simulink model "platoon"  (R2024b)
settings: Solver=FixedStepAuto  StartTime=0.0  StopTime=20  RelTol=1e-3
libraries: slpidlib x2
settings Model: Creator=Corné  LastModifiedBy=Corné

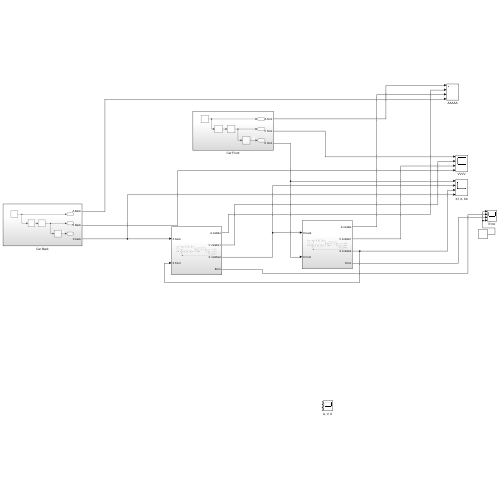
[thumbnail: Simulink's stored preview of the top-level diagram]
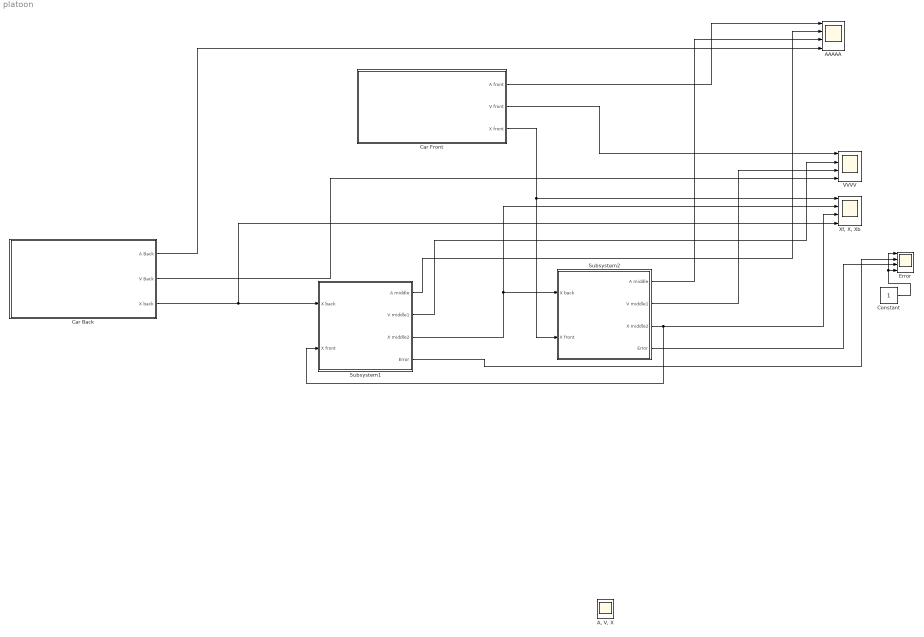
== system platoon ==
  "A, V, X " : Scope  NumInputPorts=3
  AAAAA : Scope  NumInputPorts=4
  Car Back : Subsystem
  Car Front : Subsystem
  Constant : Constant
  Error : Scope  NumInputPorts=4
  Subsystem1 : Subsystem
  Subsystem2 : Subsystem
  VVVV : Scope  NumInputPorts=4
  "Xf, X, Xb" : Scope  NumInputPorts=4
  wires:
  Car Back/3(X back) -> "Xf, X, Xb"/4, Subsystem1/1("X back ")
  Car Front/3(X front) -> Subsystem2/2(X front), "Xf, X, Xb"/1
  Subsystem1/4(Error) -> Error/2
  Subsystem1/3(X middle2) -> "Xf, X, Xb"/2, Subsystem2/1("X back ")
  Subsystem2/3(X middle2) -> "Xf, X, Xb"/3, Subsystem1/2(X front)
  Subsystem2/4(Error) -> Error/3
  Car Front/1(A front) -> AAAAA/1
  Car Back/1(A Back) -> AAAAA/4
  Subsystem1/1(A middle) -> AAAAA/2
  Subsystem2/1(A middle) -> AAAAA/3
  Car Front/2(V front) -> VVVV/1
  Car Back/2(V Back) -> VVVV/4
  Subsystem1/2(V middle1) -> VVVV/2
  Subsystem2/2(V middle1) -> VVVV/3
  Constant/1 -> Error/4, Error/1

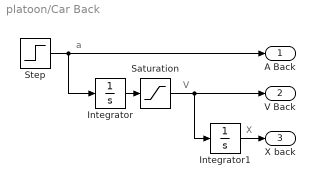
== system platoon/Car Back ==
  note: X
  note: V
  note: a
  Integrator : Integrator  InitialCondition=30
  Integrator1 : Integrator
  Saturation : Saturate  UpperLimit=30  LowerLimit=-50
  Step : Step  Time=0  After=0  SampleTime=0
  A Back : Outport
  V Back : Outport  Port=2
  X back : Outport  Port=3
  wires:
  Integrator/1 -> Saturation/1
  Step/1 -> Integrator/1, A Back/1
  Integrator1/1 -> X back/1
  Saturation/1 -> Integrator1/1, V Back/1

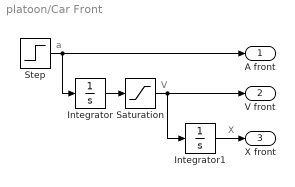
== system platoon/Car Front ==
  note: X
  note: V
  note: a
  Integrator : Integrator  InitialCondition=30
  Integrator1 : Integrator  InitialCondition=12*3
  Saturation : Saturate  UpperLimit=30  LowerLimit=-50
  Step : Step  Time=0  After=0  SampleTime=0
  A front : Outport
  V front : Outport  Port=2
  X front : Outport  Port=3
  wires:
  Integrator/1 -> Saturation/1
  Step/1 -> A front/1, Integrator/1
  Integrator1/1 -> X front/1
  Saturation/1 -> V front/1, Integrator1/1

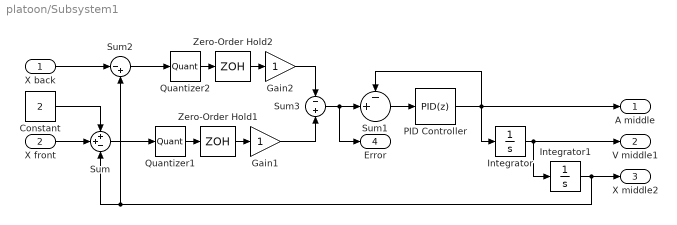
== system platoon/Subsystem1 ==
  "X back " : Inport
  X front : Inport  Port=2
  Constant : Constant  Value=2
  Gain1 : Gain
  Gain2 : Gain
  Integrator : Integrator  InitialCondition=22
  Integrator1 : Integrator  InitialCondition=10
  PID Controller : slpidlib/PID Controller  Controller=PID  Form=Parallel  TimeDomain=Discrete-time  UseExternalTs=off  SampleTime=-1  IntegratorMethod=Forward Euler  FilterMethod=Forward Euler  ControllerParametersSource=internal  P=0.2  I=0  UseKiTs=off  D=0.6  UseExternalDerivativeSource=off  N=100  UseFilter=on  TunerSelectOption=Transfer Function Based (PID Tuner App)  InitialConditionSource=internal  InitialConditionForIntegrator=0  InitialConditionForFilter=0  DifferentiatorICPrevScaledInput=0  ExternalReset=none  TrackingMode=off  Kt=1  LimitOutput=off  SatLimitsSource=internal  UpperSaturationLimit=inf  LowerSaturationLimit=-inf  LinearizeAsGain=on  AntiWindupMode=none  Kb=1  LimitIntegrator=off  UpperIntegratorSaturationLimit=inf  LowerIntegratorSaturationLimit=-inf  POutMin=[]  POutMax=[]  IOutMin=[]  IOutMax=[]  DOutMin=[]  DOutMax=[]  NOutMin=[]  NOutMax=[]  SumOutMin=[]  SumOutMax=[]  SaturationOutMin=[]  SaturationOutMax=[]  PParamMin=[]  PParamMax=[]  IParamMin=[]  IParamMax=[]  DParamMin=[]  DParamMax=[]  NParamMin=[]  NParamMax=[]  KbParamMin=[]  KbParamMax=[]  KtParamMin=[]  KtParamMax=[]  KbOutMin=[]  KbOutMax=[]  KtOutMin=[]  KtOutMax=[]  IntegratorOutMin=[]  IntegratorOutMax=[]  FilterOutMin=[]  FilterOutMax=[]  SumI1OutMin=[]  SumI1OutMax=[]  SumI2OutMin=[]  SumI2OutMax=[]  SumI3OutMin=[]  SumI3OutMax=[]  SumI4OutMin=[]  SumI4OutMax=[]  SumDOutMin=[]  SumDOutMax=[]  DifferentiatorOutMin=[]  DifferentiatorOutMax=[]  FilterDiffOutCoefMin=[]  FilterDiffOutCoefMax=[]  ReciprocalOutMin=[]  ReciprocalOutMax=[]  SumDenOutMin=[]  SumDenOutMax=[]  SumNumOutMin=[]  SumNumOutMax=[]  DivideOutMin=[]  DivideOutMax=[]  UdiffTsProdOutMin=[]  UdiffTsProdOutMax=[]  NTsProdOutMin=[]  NTsProdOutMax=[]  UintegralTsProdOutMin=[]  UintegralTsProdOutMax=[]  UngainTsProdOutMin=[]  UngainTsProdOutMax=[]  ClampingZeroOutDataTypeStr=Inherit: Inherit via back propagation  ClampingZeroOutMin=[]  ClampingZeroOutMax=[]  FilterDenConstantOutDataTypeStr=Inherit: Inherit via back propagation  FilterDenConstantOutMin=[]  FilterDenConstantOutMax=[]  PCopyOutDataTypeStr=Inherit: Inherit via back propagation  PCopyOutMin=[]  PCopyOutMax=[]  NCopyOutDataTypeStr=Inherit: Inherit via back propagation  NCopyOutMin=[]  NCopyOutMax=[]  IntegratorContinuousStateAttributes=''  IntegratorStateMustResolveToSignalObject=off  IntegratorRTWStateStorageClass=Auto  FilterContinuousStateAttributes=''  FilterStateMustResolveToSignalObject=off  FilterRTWStateStorageClass=Auto  ParallelPVariant=InternalParameters  IdealPVariant=Disabled  IVariant=InternalParameters  DVariant=InternalParameters  IntegratorVariant=Discrete  SatVariant=Disabled  AWVariant=Passthrough  PCopyVariant=Disabled  TRVariant=Disabled  FdbkBlocksVariant=Forward  IdealPFdbkVariant=Disabled  SatFdbkVariant=Disabled  DerivativeFilterVariant=ForwardEulerFilter  NVariant=InternalParameters  NCopyVariant=Disabled  FilterICVariant=InternalICsFilter  IntegratorICVariant=InternalICs  ExternalResetVariant=Disabled  TRSumVariant=Passthrough  SumFdbkVariant=Disabled  SumVariant=Sum_PID  TsampFilterVariant=InternalTs  TsampNgainVariant=Passthrough  TsampIntegralVariant=Disabled_SignalSpec  ExternalSaturationOutDataTypeStr=Inherit: Same as second input  DerivativeSourceVariant=ErrorSignal  PreIntVariant=InternalPreInt
  Quantizer1 : Quantizer  QuantizationInterval=0.1
  Quantizer2 : Quantizer  QuantizationInterval=0.1
  Sum : Sum  Inputs=++-
  Sum1 : Sum  Inputs=-+|
  Sum2 : Sum  Inputs=|-+
  Sum3 : Sum  Inputs=-|+
  Zero-Order Hold1 : ZeroOrderHold  SampleTime=0.1
  Zero-Order Hold2 : ZeroOrderHold  SampleTime=0.1
  A middle : Outport
  V middle1 : Outport  Port=2
  X middle2 : Outport  Port=3
  Error : Outport  Port=4
  wires:
  Integrator/1 -> Integrator1/1, V middle1/1
  Integrator1/1 -> Sum2/2, Sum/3, X middle2/1
  Sum1/1 -> PID Controller/1
  PID Controller/1 -> Sum1/1, Integrator/1, A middle/1
  X front/1 -> Sum/2
  Sum3/1 -> Error/1, Sum1/2
  Quantizer1/1 -> Zero-Order Hold1/1
  Zero-Order Hold1/1 -> Gain1/1
  Sum/1 -> Quantizer1/1
  Gain1/1 -> Sum3/2
  Quantizer2/1 -> Zero-Order Hold2/1
  Zero-Order Hold2/1 -> Gain2/1
  Sum2/1 -> Quantizer2/1
  Gain2/1 -> Sum3/1
  Constant/1 -> Sum/1
  "X back "/1 -> Sum2/1

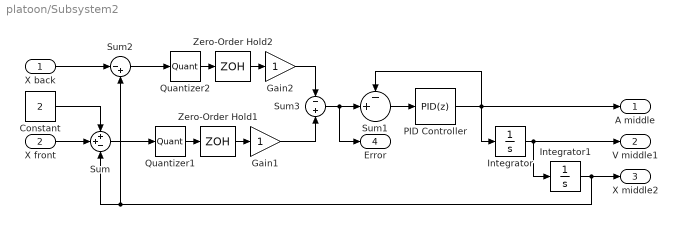
== system platoon/Subsystem2 ==
  "X back " : Inport
  X front : Inport  Port=2
  Constant : Constant  Value=2
  Gain1 : Gain
  Gain2 : Gain
  Integrator : Integrator  InitialCondition=22
  Integrator1 : Integrator  InitialCondition=20
  PID Controller : slpidlib/PID Controller  Controller=PID  Form=Parallel  TimeDomain=Discrete-time  UseExternalTs=off  SampleTime=-1  IntegratorMethod=Forward Euler  FilterMethod=Forward Euler  ControllerParametersSource=internal  P=0.2  I=0  UseKiTs=off  D=0.6  UseExternalDerivativeSource=off  N=100  UseFilter=on  TunerSelectOption=Transfer Function Based (PID Tuner App)  InitialConditionSource=internal  InitialConditionForIntegrator=0  InitialConditionForFilter=0  DifferentiatorICPrevScaledInput=0  ExternalReset=none  TrackingMode=off  Kt=1  LimitOutput=off  SatLimitsSource=internal  UpperSaturationLimit=inf  LowerSaturationLimit=-inf  LinearizeAsGain=on  AntiWindupMode=none  Kb=1  LimitIntegrator=off  UpperIntegratorSaturationLimit=inf  LowerIntegratorSaturationLimit=-inf  POutMin=[]  POutMax=[]  IOutMin=[]  IOutMax=[]  DOutMin=[]  DOutMax=[]  NOutMin=[]  NOutMax=[]  SumOutMin=[]  SumOutMax=[]  SaturationOutMin=[]  SaturationOutMax=[]  PParamMin=[]  PParamMax=[]  IParamMin=[]  IParamMax=[]  DParamMin=[]  DParamMax=[]  NParamMin=[]  NParamMax=[]  KbParamMin=[]  KbParamMax=[]  KtParamMin=[]  KtParamMax=[]  KbOutMin=[]  KbOutMax=[]  KtOutMin=[]  KtOutMax=[]  IntegratorOutMin=[]  IntegratorOutMax=[]  FilterOutMin=[]  FilterOutMax=[]  SumI1OutMin=[]  SumI1OutMax=[]  SumI2OutMin=[]  SumI2OutMax=[]  SumI3OutMin=[]  SumI3OutMax=[]  SumI4OutMin=[]  SumI4OutMax=[]  SumDOutMin=[]  SumDOutMax=[]  DifferentiatorOutMin=[]  DifferentiatorOutMax=[]  FilterDiffOutCoefMin=[]  FilterDiffOutCoefMax=[]  ReciprocalOutMin=[]  ReciprocalOutMax=[]  SumDenOutMin=[]  SumDenOutMax=[]  SumNumOutMin=[]  SumNumOutMax=[]  DivideOutMin=[]  DivideOutMax=[]  UdiffTsProdOutMin=[]  UdiffTsProdOutMax=[]  NTsProdOutMin=[]  NTsProdOutMax=[]  UintegralTsProdOutMin=[]  UintegralTsProdOutMax=[]  UngainTsProdOutMin=[]  UngainTsProdOutMax=[]  ClampingZeroOutDataTypeStr=Inherit: Inherit via back propagation  ClampingZeroOutMin=[]  ClampingZeroOutMax=[]  FilterDenConstantOutDataTypeStr=Inherit: Inherit via back propagation  FilterDenConstantOutMin=[]  FilterDenConstantOutMax=[]  PCopyOutDataTypeStr=Inherit: Inherit via back propagation  PCopyOutMin=[]  PCopyOutMax=[]  NCopyOutDataTypeStr=Inherit: Inherit via back propagation  NCopyOutMin=[]  NCopyOutMax=[]  IntegratorContinuousStateAttributes=''  IntegratorStateMustResolveToSignalObject=off  IntegratorRTWStateStorageClass=Auto  FilterContinuousStateAttributes=''  FilterStateMustResolveToSignalObject=off  FilterRTWStateStorageClass=Auto  ParallelPVariant=InternalParameters  IdealPVariant=Disabled  IVariant=InternalParameters  DVariant=InternalParameters  IntegratorVariant=Discrete  SatVariant=Disabled  AWVariant=Passthrough  PCopyVariant=Disabled  TRVariant=Disabled  FdbkBlocksVariant=Forward  IdealPFdbkVariant=Disabled  SatFdbkVariant=Disabled  DerivativeFilterVariant=ForwardEulerFilter  NVariant=InternalParameters  NCopyVariant=Disabled  FilterICVariant=InternalICsFilter  IntegratorICVariant=InternalICs  ExternalResetVariant=Disabled  TRSumVariant=Passthrough  SumFdbkVariant=Disabled  SumVariant=Sum_PID  TsampFilterVariant=InternalTs  TsampNgainVariant=Passthrough  TsampIntegralVariant=Disabled_SignalSpec  ExternalSaturationOutDataTypeStr=Inherit: Same as second input  DerivativeSourceVariant=ErrorSignal  PreIntVariant=InternalPreInt
  Quantizer1 : Quantizer  QuantizationInterval=0.1
  Quantizer2 : Quantizer  QuantizationInterval=0.1
  Sum : Sum  Inputs=++-
  Sum1 : Sum  Inputs=-+|
  Sum2 : Sum  Inputs=|-+
  Sum3 : Sum  Inputs=-|+
  Zero-Order Hold1 : ZeroOrderHold  SampleTime=0.1
  Zero-Order Hold2 : ZeroOrderHold  SampleTime=0.1
  A middle : Outport
  V middle1 : Outport  Port=2
  X middle2 : Outport  Port=3
  Error : Outport  Port=4
  wires:
  Integrator/1 -> Integrator1/1, V middle1/1
  Integrator1/1 -> Sum2/2, Sum/3, X middle2/1
  Sum1/1 -> PID Controller/1
  PID Controller/1 -> Sum1/1, Integrator/1, A middle/1
  X front/1 -> Sum/2
  Sum3/1 -> Error/1, Sum1/2
  Quantizer1/1 -> Zero-Order Hold1/1
  Zero-Order Hold1/1 -> Gain1/1
  Sum/1 -> Quantizer1/1
  Gain1/1 -> Sum3/2
  Quantizer2/1 -> Zero-Order Hold2/1
  Zero-Order Hold2/1 -> Gain2/1
  Sum2/1 -> Quantizer2/1
  Gain2/1 -> Sum3/1
  Constant/1 -> Sum/1
  "X back "/1 -> Sum2/1
